simulink model "continuum0513"  (R2020a)
settings: Solver=VariableStepAuto  StartTime=0.0  StopTime=inf  RelTol=1e-3
settings Model: Creator=Vulca  LastModifiedBy=Vulca
settings ConfigComp: DVTestSuiteOptimization=Auto  DVDetectOutOfBounds=on

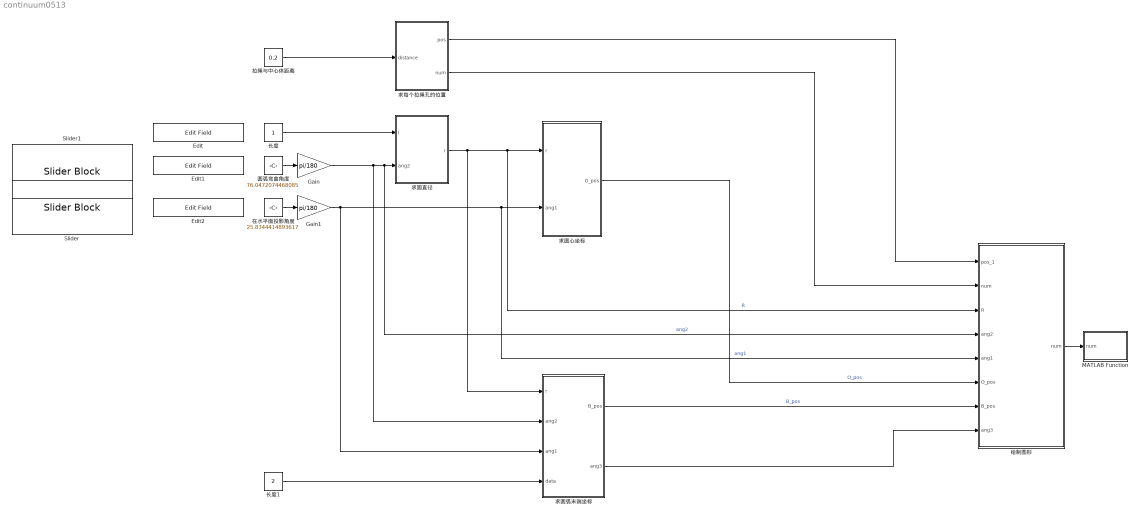
== system continuum0513 ==
  Edit : EditField  LabelPosition=Hide  ShowInitialText=on  Alignment=Center
  Edit1 : EditField  LabelPosition=Hide  ShowInitialText=on  Alignment=Center
  Edit2 : EditField  LabelPosition=Hide  ShowInitialText=on  Alignment=Center
  Gain : Gain  Gain=pi/180
  Gain1 : Gain  Gain=pi/180
  MATLAB Function : MATLAB Function  TreatAsAtomicUnit=on
  Slider : SliderBlock
  Slider1 : SliderBlock
  圆弧弯曲角度 : Constant  Value=76.0472074468085
  在水平面投影角度 : Constant  Value=25.8344414893617
  拉绳与中心体距离 : Constant  Value=0.2
  求圆弧末端坐标 : MATLAB Function  TreatAsAtomicUnit=on
  求圆心坐标 : MATLAB Function  TreatAsAtomicUnit=on
  求圆直径 : MATLAB Function  TreatAsAtomicUnit=on
  求每个拉绳孔的位置 : MATLAB Function  TreatAsAtomicUnit=on
  绘制图形 : MATLAB Function  TreatAsAtomicUnit=on  VariantControl=Choice
  长度 : Constant
  长度1 : Constant  Value=2
  wires:
  长度/1 -> 求圆直径/1(l)
  圆弧弯曲角度/1 -> Gain/1
  在水平面投影角度/1 -> Gain1/1
  求圆直径/1(r) -> 绘制图形/3(R), 求圆心坐标/1(r), 求圆弧末端坐标/1(r)  "R"
  Gain/1 -> 绘制图形/4(ang2), 求圆直径/2(ang2), 求圆弧末端坐标/2(ang2)  "ang2"
  Gain1/1 -> 绘制图形/5(ang1), 求圆心坐标/2(ang1), 求圆弧末端坐标/3(ang1)  "ang1"
  拉绳与中心体距离/1 -> 求每个拉绳孔的位置/1(distance)
  求每个拉绳孔的位置/1(pos) -> 绘制图形/1(pos_1)
  求每个拉绳孔的位置/2(num) -> 绘制图形/2("num ")
  求圆心坐标/1(O_pos) -> 绘制图形/6(O_pos)  "O_pos"
  求圆弧末端坐标/1(B_pos) -> 绘制图形/7(B_pos)  "B_pos"
  求圆弧末端坐标/2(ang3) -> 绘制图形/8(ang3)
  绘制图形/1(num) -> MATLAB Function/1(num)
  长度1/1 -> 求圆弧末端坐标/4(data)

== matlab function continuum0513/求圆心坐标 ==
  data: r input; O_pos output; ang1 input
function O_pos = fcn(r,ang1)
    %计算X坐标
    x = r * cos(ang1);
    %计算Y坐标
    y = r * sin(ang1);
    
    O_pos = [x,y,0];
end

== matlab function continuum0513/求圆直径 ==
  data: l input; r output; ang2 input
function r = fcn(l,ang2)
    %将ang2转换为弧度制
    double ang2_degree;
    ang2_degree = ang2;
    %计算半径
    r = l/ang2_degree;
end

== matlab function continuum0513/求圆弧末端坐标 ==
  data: r input; B_pos output; ang2 input; ang1 input; ang3 output; data input
function [B_pos,ang3]  = fcn(r,ang2,ang1, data)
double L;
double Lob;
%定义盘片坐标数组
num = 3;
B_pos = zeros(num,3);
pos = zeros(1,3);
%计算每个盘片的坐标
for index = 1:1:data
     %B点Z轴坐标
     z = r * sin(ang2 * index/data);
     %B点X轴坐标
     x = r - r * cos(ang2 * index/data);
     %B点整体坐标
     pos =[x 0 z];
     %计算弦长
     L = 2 * r * sin(ang2 * index /data  / 2);
     %B点投影于XOY平面AB的长度
     Lob = L * cos ((pi - ang2)/2);
     %B点X轴坐标-Lob投影于X轴的长度
     x = Lob* cos(ang1);
     %B点Y轴坐标-Lob投影于Y轴的长度
     y = Lob* sin(ang1);
end
   %B点坐标
    B_pos; % = [x,y,z];
    %计算B点在XOZ平面内的角度偏转
    ang3 = 2 * (pi/2 - (pi - ang2)/2);
end

== matlab function continuum0513/MATLAB Function ==
  data: num input
function fcn(num)
    axis equal;
    xlabel('x');
    ylabel('y');
    zlabel('z');
    xlim([-1 1]); 
    ylim([-1 1]);
    zlim([0 2]);
    grid on;
end

== matlab function continuum0513/求每个拉绳孔的位置 ==
  data: distance input; pos output; num output
function [pos,num]  = fcn(distance)
    %线数目
    num = 3;
    %定义pos
    pos = zeros (num,3);
    %计算间隔角度
    degree_1 = 2*pi/num;
    %使用三角函数计算坐标
    for index = 1:num
        pos(index,1) = distance * cos(degree_1*index);
        pos(index,2) = distance * sin(degree_1*index);
        pos(index,3) = 0;
    end
end

== matlab function continuum0513/绘制图形 ==
  data: pos_1 input; num input; R input; ang2 input; ang1 input; O_pos input; B_pos input; ang3 input; num output
function num = fcn(pos_1, num, R, ang2,ang1,O_pos,B_pos, ang3)
    %清除
    clf;
    %表格配置，轴对齐
    %axis manual;
    
    %绘制A点
    plot3(0,0,0,'o');
    hold on;
    %绘制B点
    plot3(B_pos(1),B_pos(2),B_pos(3),'o','color','r');
    text(B_pos(1),B_pos(2),B_pos(3),'B');
    hold on;
    %绘制O点-圆心
    plot3(O_pos(1),O_pos(2),O_pos(3),'o','color','g');
    text(O_pos(1),O_pos(2),O_pos(3),'O');
    %绘制A点-起点
    plot3(0,0,0,'o','color','y');
    text(0,0,0,'A');
    hold on;
    %绘制直线AB
    plot3([0,B_pos(1)],[0,B_pos(2)],[0,B_pos(3)],'--');
    hold on;
    %计算第一个旋转矩阵
    N = rotz(ang1*180/pi);
    M = rotz(ang1*180/pi);
    %计算空间圆弧上的点每一个点的X坐标,Y坐标和Z坐标
    ang2_array = linspace(0,ang2,50);
    double point_arc_x;
    point_arc_x = linspace(0,0,50);
    double point_arc_y;
    point_arc_y = linspace(0,0,50);
    double point_arc_z;
    point_arc_z = linspace(0,0,50);
    for index = 1:1:50
        point_arc_x(index) =  R-R * cos(ang2_array(index));
        point_arc_y(index) =  0;
        point_arc_z(index) =  R * sin(ang2_array(index));
        point = ([point_arc_x(index),point_arc_y(index),point_arc_z(index)]);
        point2 = (N * point');
        point_arc_x(index) = point2(1);
        point_arc_y(index) = point2(2);
        point_arc_z(index) = point2(3);
    end
    %绘制圆弧
    plot3(point_arc_x,point_arc_y,point_arc_z);
    %计算第二个旋转矩阵
    M = angvec2r(ang3,N*[0 1 0]');
    
    %绘制拉绳孔
    for index = 1:num
        point3 = pos_1(index,1:3)';
        point4 = M * point3 + B_pos';
        plot3([point3(1),0],[point3(2),0],[point3(3),0],'black');
        plot3([point4(1),B_pos(1)],[point4(2),B_pos(2)],[point4(3),B_pos(3)],'black');
        plot3([point4(1),point3(1)],[point4(2),point3(2)],[point4(3),point3(3)],'g--');
    end
end
